simulink model "IMC_Simulink"  (R2018b)
settings: Solver=VariableStepAuto  StartTime=0.0  StopTime=5  RelTol=1e-3
values from neighbouring files (symbols this model uses):
  Kc = vars(5)    [Optimum.m]
  N = vars(4)    [CC.m]    (also in CHR.m; Optimum.m; PID_1.m = 10; PID_10.m = 10)
  Td = ((0.27-0.36*tau)/(1-0.87*tau)) * L    [CC.m]    (also in CHR.m = KK(typ, 6) * L; FOIPDT.m = T; IPDT.m = a(iC, 5) * L; Optimum.m = 0.144 * Tc)
  Ti = ((2.5-2*tau)/(1-0.39*tau)) * L    [CC.m]    (also in CHR.m = KK(typ, 5) * TT; FOIPDT.m = 2 * L * (1+a); IPDT.m = a(iC, 4) * L; Optimum.m = Tc * (1.751*kappa-0.612) / (3.776*kappa+1.388))
undefined symbols (not defined in the file or in its folder): b, c, Nsat
settings Model: Creator=Erfan Etesami  LastModifiedBy=Erfan Etesami

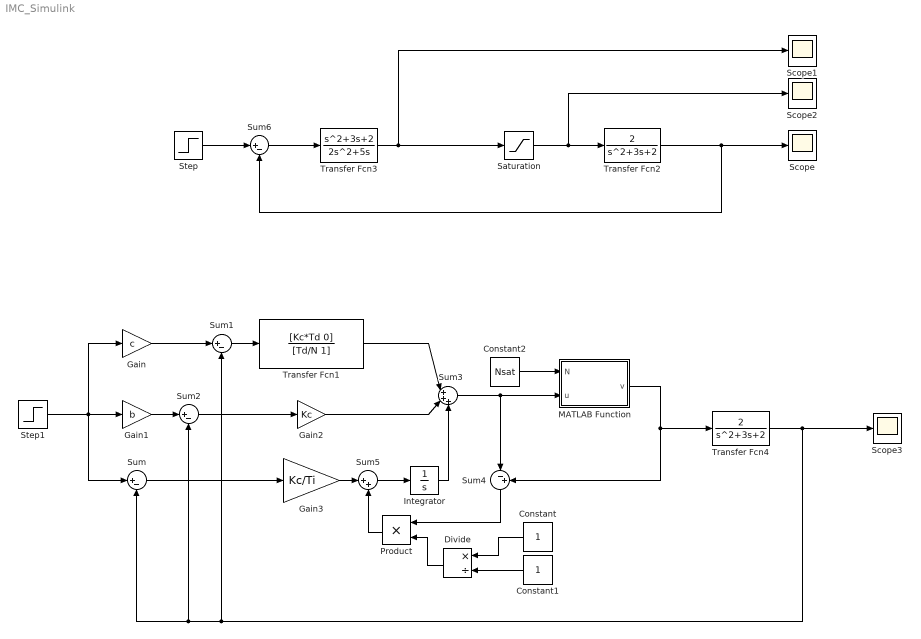
== system IMC_Simulink ==
  Constant : Constant
  Constant1 : Constant
  Constant2 : Constant  Value=Nsat
  Divide : Product  Inputs=*/
  Gain : Gain  Gain=c
  Gain1 : Gain  Gain=b
  Gain2 : Gain  Gain=Kc
  Gain3 : Gain  Gain=Kc/Ti
  Integrator : Integrator
  MATLAB Function : MATLAB Function  TreatAsAtomicUnit=on
  Product : Product
  Saturation : Saturate  UpperLimit=Nsat  LowerLimit=-Nsat
  Scope{,1..3} (4 alike) : Scope
  Step : Step  Time=0  SampleTime=0
  Step1 : Step  Time=0  SampleTime=0
  Sum{,1..2,6} (4 alike) : Sum  Inputs=|+-
  Sum3 : Sum  Inputs=|+++
  Sum4 : Sum  Inputs=|-+
  Sum5 : Sum  Inputs=|++
  Transfer Fcn1 : TransferFcn  Numerator=[Kc*Td 0]  Denominator=[Td/N 1]
  Transfer Fcn2 : TransferFcn  Numerator=[2]  Denominator=[1 3 2]
  Transfer Fcn3 : TransferFcn  Numerator=[1 3 2]  Denominator=[2 5 0]
  Transfer Fcn4 : TransferFcn  Numerator=[2]  Denominator=[1 3 2]
  wires:
  Constant2/1 -> MATLAB Function/1(N)
  Gain3/1 -> Sum5/1
  Gain/1 -> Sum1/1
  Gain1/1 -> Sum2/1
  Product/1 -> Sum5/2
  MATLAB Function/1(v) -> Transfer Fcn4/1, Sum4/2
  Sum1/1 -> Transfer Fcn1/1
  Integrator/1 -> Sum3/3
  Sum4/1 -> Product/1
  Sum5/1 -> Integrator/1
  Sum3/1 -> MATLAB Function/2(u), Sum4/1
  Step1/1 -> Gain/1, Sum/1, Gain1/1
  Constant1/1 -> Divide/2
  Sum/1 -> Gain3/1
  Transfer Fcn1/1 -> Sum3/1
  Gain2/1 -> Sum3/2
  Constant/1 -> Divide/1
  Transfer Fcn4/1 -> Scope3/1, Sum1/2, Sum2/2, Sum/2
  Sum2/1 -> Gain2/1
  Divide/1 -> Product/2
  Step/1 -> Sum6/1
  Sum6/1 -> Transfer Fcn3/1
  Transfer Fcn2/1 -> Sum6/2, Scope/1
  Transfer Fcn3/1 -> Saturation/1, Scope1/1
  Saturation/1 -> Transfer Fcn2/1, Scope2/1

== matlab function IMC_Simulink/MATLAB Function ==
  data: N input; u input; v output
function v = fcn(N, u)

v = min(N, max(-N, u));

end
